simulink model "SimulinkModel_Template"  (Simulink 7.9)
settings: Solver=FixedStepDiscrete  SolverMode=MultiTasking  StartTime=0.0  StopTime=RunningTime  FixedStep=sample  RelTol=1e-3
values from neighbouring files (symbols this model uses):
  Integrator = CreateIntegrator(data(4), data(5), data(6), data2(1), data2(2))    [LoadConfiguration.m]    (also in ModelSetup.m = InitializeIntegrator(Integrator, Structure))
  NumFreeDOF = Structure.NumFreeDOF    [ModelSetup.m]
  RigidLinkMasterMatrix = Structure.RigidLinkMasterMatrix    [ModelSetup.m]
  RigidLinkNo = Structure.RigidLinkNo    [ModelSetup.m]
  RigidLinkNodeID = Structure.RigidLinkNodeID    [ModelSetup.m]
  RigidLinkSlaveMatrix = Structure.RigidLinkSlaveMatrix    [ModelSetup.m]
  sample = SampleRate/Integrator.Interpolations    [ModelSetup.m]
  SampleRate = Integrator.Timestep    [ModelSetup.m]
  Structure = CalculateMatrices(Structure, Elements, Integrator)    [ModelSetup.m]
undefined symbols (not defined in the file or in its folder): ElementsStruct
libraries: simulink x2
(part 1 of 2)
CloseFcn:
  | rtwprivate ssgencode ModelCloseRequest hybriddaq1dof
settings Model: MinMaxOverflowLogging=ForceOff  Creator=RTMD  LastModifiedBy=Thomas Marullo  BufferReuse=off
settings DataIOCC: LimitDataPoints=off
settings OptimizationCC: BlockReduction=off  OptimizeBlockIOStorage=off  BufferReuse=off  ExpressionFolding=off  LocalBlockOutputs=off  InitFltsAndDblsToZero=on
settings DebuggingCC: SignalResolutionControl=TryResolveAllWithWarning  MultiTaskDSMMsg=warning  FcnCallInpInsideContextMsg=Use local settings
settings HardwareCC: ProdIntDivRoundTo=Zero  ProdEndianess=LittleEndian  ProdHWDeviceType=Generic->32-bit x86 compatible
settings SFSimCC: SimParseCustomCode=off
settings RTWCC: ProcessScript=grt_make_rtw_hook  RTWCompilerOptimization=On
settings GRTTargetCC: CombineOutputUpdateFcns=off  GRTInterface=on

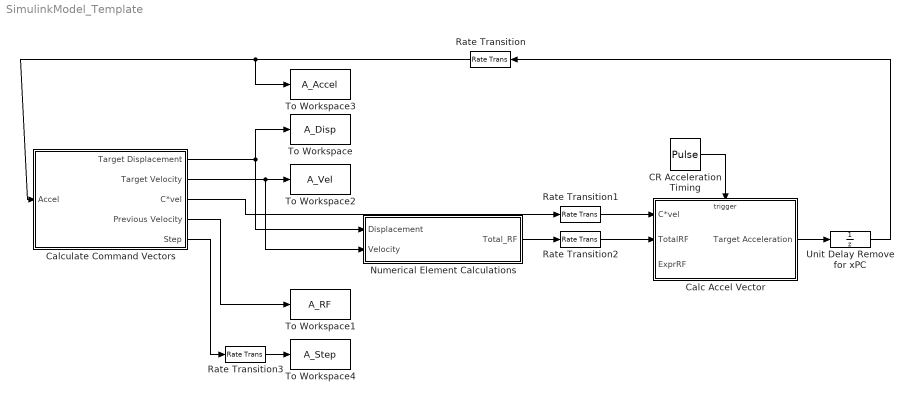
== system SimulinkModel_Template ==
  CR Acceleration Timing : DiscretePulseGenerator  Period=Integrator.Interpolations  PhaseDelay=Integrator.Interpolations-1  SampleTime=sample
  Calc Accel Vector : Subsystem
  Calculate Command Vectors : Subsystem  TreatAsAtomicUnit=on  SystemSampleTime=SampleRate
  Numerical Element Calculations : MATLAB Function  TreatAsAtomicUnit=on
  Rate Transition : RateTransition  Deterministic=off  OutPortSampleTime=SampleRate
  Rate Transition1 : RateTransition  Deterministic=off  OutPortSampleTime=sample
  Rate Transition2 : RateTransition  Deterministic=off  OutPortSampleTime=sample
  Rate Transition3 : RateTransition  Deterministic=off  OutPortSampleTime=sample
  To Workspace : ToWorkspace  VariableName=A_Disp  SampleTime=-1
      settings: MaxDataPoints=Integrator.Steps
  To Workspace1 : ToWorkspace  VariableName=A_RF  SampleTime=-1
      settings: MaxDataPoints=Integrator.Steps
  To Workspace2 : ToWorkspace  VariableName=A_Vel  SampleTime=-1
      settings: MaxDataPoints=Integrator.Steps
  To Workspace3 : ToWorkspace  VariableName=A_Accel  SampleTime=-1
      settings: MaxDataPoints=Integrator.Steps
  To Workspace4 : ToWorkspace  VariableName=A_Step  SampleTime=-1
      settings: MaxDataPoints=Integrator.Steps
  Unit Delay Remove for xPC : UnitDelay  SampleTime=-1
  wires:
  CR Acceleration Timing/1 -> Calc Accel Vector/Trigger
  Calculate Command Vectors/4(Previous Velocity) -> To Workspace1/1
  Calc Accel Vector/1(Target Acceleration) -> Unit Delay Remove for xPC/1
  Calculate Command Vectors/1(Target Displacement) -> To Workspace/1, Numerical Element Calculations/1(Displacement)
  Rate Transition/1 -> Calculate Command Vectors/1(Accel), To Workspace3/1
  Calculate Command Vectors/2(Target Velocity) -> To Workspace2/1, Numerical Element Calculations/2(Velocity)
  Calculate Command Vectors/5(Step) -> Rate Transition3/1
  Unit Delay Remove for xPC/1 -> Rate Transition/1
  Rate Transition3/1 -> To Workspace4/1
  Rate Transition1/1 -> Calc Accel Vector/1(C*vel)
  Rate Transition2/1 -> Calc Accel Vector/2(TotalRF)
  Numerical Element Calculations/1(Total_RF) -> Rate Transition2/1
  Calculate Command Vectors/3(C*vel) -> Rate Transition1/1

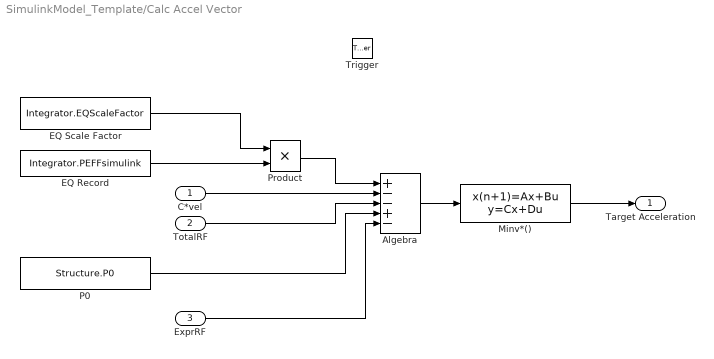
== system SimulinkModel_Template/Calc Accel Vector ==
  C*vel : Inport
  TotalRF : Inport  Port=2
  ExprRF : Inport  Port=3
  Trigger : TriggerPort
  Algebra : Sum  Inputs=+--+-
  EQ Record : FromWorkspace  VariableName=Integrator.PEFFsimulink  Interpolate=off  OutputAfterFinalValue=Holding final value
  EQ Scale Factor : Constant  Value=Integrator.EQScaleFactor
  Minv*() : DiscreteStateSpace  A=[]  B=[]  C=[]  D=Structure.MassMatrixFreeInv  SampleTime=-1
  P0 : Constant  Value=Structure.P0
  Product : Product  RndMeth=Zero
  Target Acceleration : Outport
  wires:
  TotalRF/1 -> Algebra/3
  P0/1 -> Algebra/4
  Algebra/1 -> Minv*()/1
  Product/1 -> Algebra/1
  EQ Scale Factor/1 -> Product/1
  EQ Record/1 -> Product/2
  C*vel/1 -> Algebra/2
  Minv*()/1 -> Target Acceleration/1
  ExprRF/1 -> Algebra/5

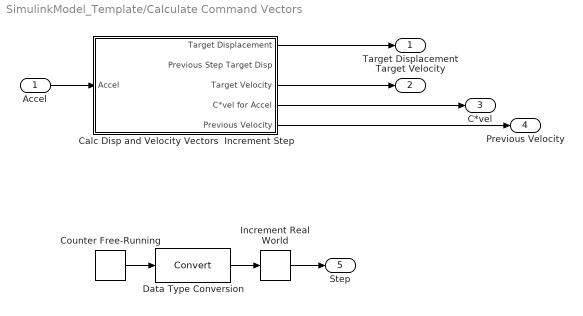
== system SimulinkModel_Template/Calculate Command Vectors ==
  Accel : Inport
  Calc Disp and Velocity Vectors  Increment Step : Subsystem
  Counter Free-Running : simulink/Sources/Counter Free-Running  NumBits=16  tsamp=-1
  Data Type Conversion : DataTypeConversion
  Increment Real World : simulink/Additional Math & Discrete/Additional Math: Increment - Decrement/Increment Real World
  Target Displacement : Outport
  Target Velocity : Outport  Port=2
  C*vel : Outport  Port=3
  Previous Velocity : Outport  Port=4  InitialOutput=Integrator.RestoringForce
  Step : Outport  Port=5  InitialOutput=Integrator.RestoringForce
  wires:
  Calc Disp and Velocity Vectors  Increment Step/1(Target Displacement) -> Target Displacement/1
  Calc Disp and Velocity Vectors  Increment Step/3(Target Velocity) -> Target Velocity/1
  Calc Disp and Velocity Vectors  Increment Step/4(C*vel for Accel) -> C*vel/1
  Accel/1 -> Calc Disp and Velocity Vectors  Increment Step/1(Accel)
  Counter Free-Running/1 -> Data Type Conversion/1
  Data Type Conversion/1 -> Increment Real World/1
  Increment Real World/1 -> Step/1
  Calc Disp and Velocity Vectors  Increment Step/5(Previous Velocity) -> Previous Velocity/1

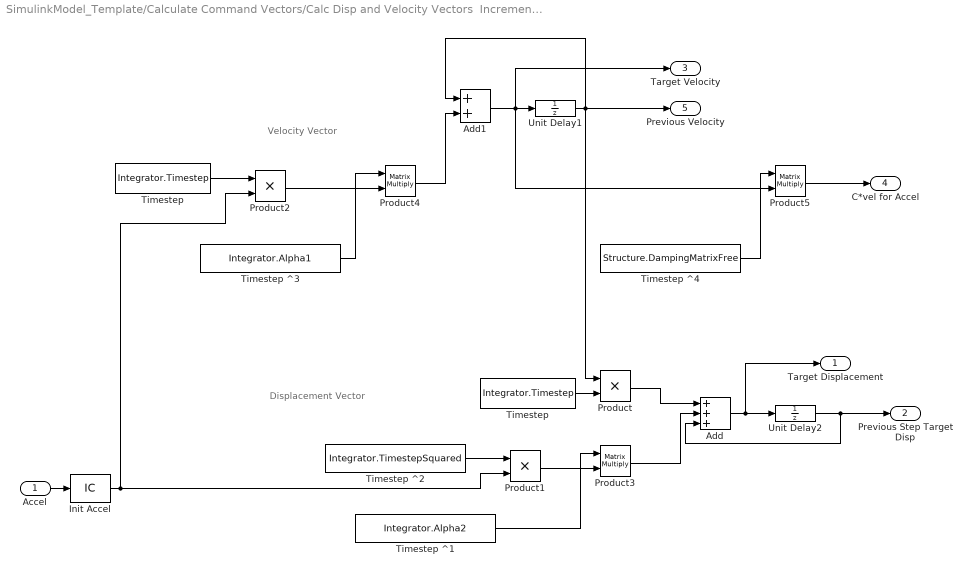
== system SimulinkModel_Template/Calculate Command Vectors/Calc Disp and Velocity Vectors  Increment Step ==
  note: Velocity Vector
  note: Displacement Vector
  Accel : Inport
  Add : Sum  Inputs=+++
  Add1 : Sum
  Init Accel : InitialCondition  Value=Integrator.Acceleration
  Product : Product  RndMeth=Zero
  Product1 : Product  RndMeth=Zero
  Product2 : Product  RndMeth=Zero
  Product3 : Product  Multiplication=Matrix(*)  RndMeth=Zero
  Product4 : Product  Multiplication=Matrix(*)  RndMeth=Zero
  Product5 : Product  Multiplication=Matrix(*)  RndMeth=Zero
  Timestep : Constant  Value=Integrator.Timestep
  "Timestep " : Constant  Value=Integrator.Timestep
  Timestep ^1 : Constant  Value=Integrator.Alpha2
  Timestep ^2 : Constant  Value=Integrator.TimestepSquared
  Timestep ^3 : Constant  Value=Integrator.Alpha1
  Timestep ^4 : Constant  Value=Structure.DampingMatrixFree
  Unit Delay1 : UnitDelay  SampleTime=-1
  Unit Delay2 : UnitDelay  SampleTime=-1
  Target Displacement : Outport
  Previous Step Target Disp : Outport  Port=2
  Target Velocity : Outport  Port=3
  C*vel for Accel : Outport  Port=4
  Previous Velocity : Outport  Port=5
  wires:
  Add/1 -> Unit Delay2/1, Target Displacement/1
  Product1/1 -> Product3/2
  Accel/1 -> Init Accel/1
  Timestep ^2/1 -> Product1/1
  Add1/1 -> Unit Delay1/1, Target Velocity/1, Product5/2
  "Timestep "/1 -> Product2/1
  Product2/1 -> Product4/2
  Timestep/1 -> Product/2
  Product/1 -> Add/1
  Product3/1 -> Add/2
  Unit Delay2/1 -> Add/3, Previous Step Target Disp/1
  Unit Delay1/1 -> Add1/1, Product/1, Previous Velocity/1
  Timestep ^1/1 -> Product3/1
  Product4/1 -> Add1/2
  Timestep ^3/1 -> Product4/1
  Product5/1 -> C*vel for Accel/1
  Timestep ^4/1 -> Product5/1
  Init Accel/1 -> Product1/2, Product2/2
